simulink model "sample_physmod_load"  (Simulink 6.4)
settings: Solver=ode23tb  StartTime=0.0  StopTime=10.0  RelTol=1e-3
libraries: driveline x5, dc_motor_lib x1
settings Model: LastModifiedBy=roaa

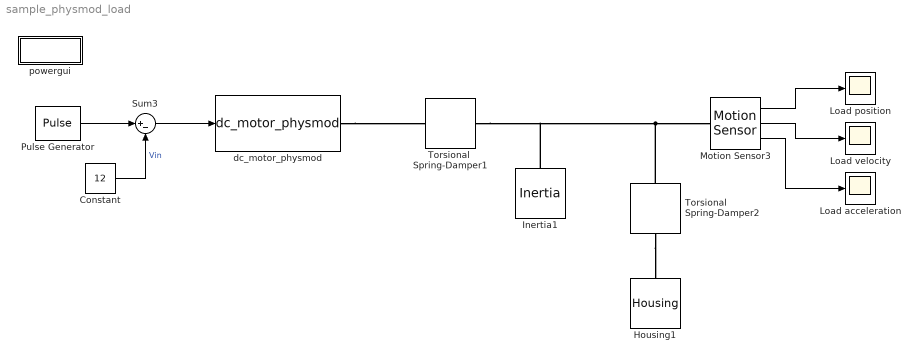
== system sample_physmod_load ==
  Constant : Constant  Value=12  OutDataType=sfix(16)  ConRadixGroup=Use specified scaling  OutScaling=2^0  SampleTime=inf  FramePeriod=inf
  Housing1 : driveline/Solver & Inertias/Housing  Orientation=up  SystemSampleTime=-1
  Inertia1 : driveline/Solver & Inertias/Inertia  Orientation=up  SystemSampleTime=-1  PortType=p1  BlockClass=Inertia  PhysicalDomain=driveline_domain  I=10.07e-6  Ip=[]  Iv=[]  ShowLeft=off  ShowRight=on
  Load acceleration : Scope
  Load position : Scope
      settings: SaveName=ScopeData3
  Load velocity : Scope
  Motion Sensor3 : driveline/Sensors & Actuators/Motion Sensor  SystemSampleTime=-1  Angle=on  x0=0  Velocity=on  Acceleration=on
  Pulse Generator : DiscretePulseGenerator  PulseType=Time based  Amplitude=24  Period=10  PulseWidth=50
  Sum3 : Sum  Inputs=|+-
  Torsional  Spring-Damper1 : driveline/Dynamic Elements/Torsional  Spring-Damper  SystemSampleTime=-1  k=100  c=0.0001  x0=0  Backlash=0
  Torsional  Spring-Damper2 : driveline/Dynamic Elements/Torsional  Spring-Damper  Orientation=up  SystemSampleTime=-1  k=0  c=12e-6  x0=0  Backlash=0
  dc_motor_physmod : dc_motor_lib/dc_motor_physmod  SystemSampleTime=-1  Rm=2.06  Lm=0.000238  Kb=1/((406*2*pi)/60)  Kt=0.0235  Jm=1.07e-6  bm=12e-7
  powergui : Subsystem  AncestorBlock=powerlib/powergui  InitFcn=|  mask(PSB option menu block){SimulationMode=Continuous, SampleTime=0, echomessages=off, x0status=blocks, Frange=[0:2:500], Ylog=off, Xlog=on, ShowGrid=off, save=off, variable=ZData, structure=, ZoomFFT=on, StartTime=0.0, cycles=1, DisplayStyle=1, fundamental=60, FreqAxis=off, MaxFrequency=1000, frequencyindice=1, frequencyindicesteady=1, RmsSteady=1, display=off, Ts=0, frequency=60, methode=off}
      | powerguiblock = gcb;                                        
      | blk = get_param(powerguiblock,'blocks');                    
      | NbBlocks = length(blk);                                     
      | if NbBlocks>2                                               
      | % clean-up:                                                 
      | for m=1:NbBlocks-2                                          
      | delete_block([powerguiblock,'/EquivalentModel',num2str(m)]);
      | end                                                         
      | end
      mask prompts: SimulationMode "General parameter: Simulation Mode"; SampleTime "General parameter: Sample Time"; echomessages "General parameter: Echo  Messages"; x0status "Initial electrical states status"; Frange "Impedance tool: Frequency Range"; Ylog "Impedance tool: Log impedance"; Xlog "Impedance tool: log Frequency"; ShowGrid "Impedance tool: grid"; save "Impedance tool: Save Data To Workspace"; variable "Impedance tool: Variable Name"; structure "Structure Name (PSBFFTSCOPE)"; ZoomFFT "ZoomFFT (PSBFFTSCOPE)"; StartTime "Start Time (PSBFFTSCOPE)"; cycles "Cycles (PSBFFTSCOPE)"; DisplayStyle "Display style (PSBFFTSCOPE)"; fundamental "Fundamental (PSBFFTSCOPE)"; FreqAxis "Frequency Axis (PSBFFTSCOPE)"; MaxFrequency "Max Frequency (PSBFFTSCOPE)"; frequencyindice "Frequency indice  (PSBLOADFLOW)"; frequencyindicesteady "Frequency indice (STEADYSTATE)"; RmsSteady "RMS display (STEADYSTATE)"; display "Display Results"; Ts "Sample time (s):"; frequency "General parameter: phasor frequency"; methode "Phasor simulation"
      mask init:
      | powerlibroot = which('powersysdomain');
      | PSBroot = powerlibroot(1:end-16);
      | %
      | switch SimulationMode
      | 	case 1
      | 		message=sprintf('Continuous');
      | 	case 2
      |         message=sprintf('Discrete,\nTs = %.4g s.',SampleTime);
      | 	case 3
      | 		message=sprintf('Phasors');
      | end
      | if strcmp(bdroot,'powerlib')
      |   message='powergui';
      | end
      | power_initmask();
      settings: CopyFcn=powergui('Copy_Callback',gcb,0,[]);  DeleteFcn=powergui('Copy_Callback',gcb,1,[]);powergui('Close_Callback',gcb,[],[]);  ModelCloseFcn=powergui('Close_Callback',gcb,[],[]);  NameChangeFcn=handles = get_param(gcb,'UserData');if ~isempty(handles);delete(handles.powergui);end
      settings: PreSaveFcn=|
      | %try
      | %close(get_param(gcbh,'userdata'))
      | %end
      | 
      | powergui('Close_Callback',gcb,[],[]);
      settings: OpenFcn=|
      | if (power_openblockproxy ('secondary'))
      | powergui(gcb,'PM')
      | end;
      mask Help: web(psbhelp)
      mask StyleString: popup(Continuous|Discrete|Phasor),edit,checkbox,popup(blocks|steady|zero),edit,checkbox,checkbox,checkbox,checkbox,edit,edit,checkbox,edit,edit,edit,edit,checkbox,edit,edit,edit,edit,checkbox,edit,edit,checkbox
      mask Display: disp(message)
  wires:
  Pulse Generator/1 -> Sum3/1
  Constant/1 -> Sum3/2  "Vin"
  Sum3/1 -> dc_motor_physmod/1
  Motion Sensor3/1 -> Load position/1
  Motion Sensor3/2 -> Load velocity/1
  Motion Sensor3/3 -> Load acceleration/1
  connections:
  dc_motor_physmod/RConn1 -- Torsional  Spring-Damper1/LConn1
  Torsional  Spring-Damper2/LConn1 -- Housing1/RConn1
  Torsional  Spring-Damper1/RConn1 -- Inertia1/RConn1 -- Motion Sensor3/LConn1 -- Torsional  Spring-Damper2/RConn1

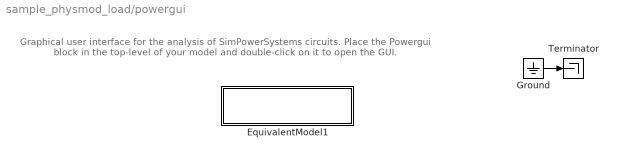
== system sample_physmod_load/powergui ==
  note: Graphical user interface for the analysis of  SimPowerSystems circuits.
      | Place the Powergui block in the top-level of your model and double-click
      | on it to open the GUI.
  EquivalentModel1 : Subsystem
      mask init:
      | SPS = get_param(gcbh,'UserData');
      | if isempty(SPS)
      |     A=0;
      |     B=0;
      |     C=0;
      |     D=0;
      |     x0=0;
      | else
      | 	A=SPS.A;
      |     B=SPS.B;
      |     C=SPS.C;
      |     D=SPS.D;
      |     x0=SPS.x0;
      | end
      mask Display:
      | color('green')
      | disp('EQUIVALENT CIRCUIT')
  Ground : Ground
  Terminator : Terminator
  wires:
  Ground/1 -> Terminator/1

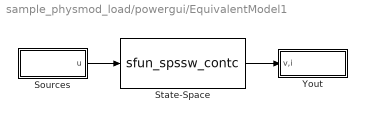
== system sample_physmod_load/powergui/EquivalentModel1 ==
  Sources : Subsystem
  State-Space : S-Function  FunctionName=sfun_spssw_contc  Parameters=A, B, C, D, x0
  Yout : Subsystem
  wires:
  State-Space/1 -> Yout/1(v,i)
  Sources/1(u) -> State-Space/1

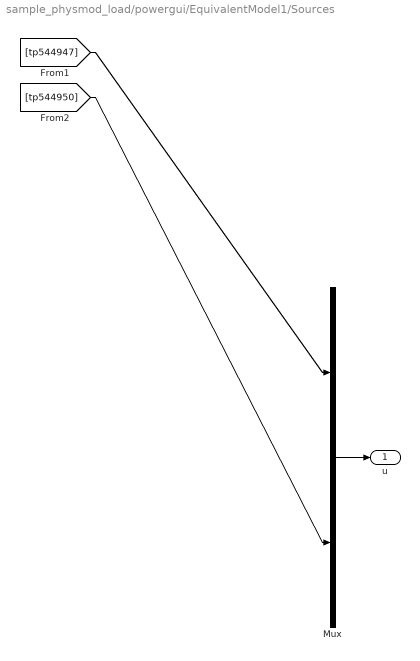
== system sample_physmod_load/powergui/EquivalentModel1/Sources ==
  Mux : Mux  Inputs=[1 1]
  u : Outport
  wires:
  Mux/1 -> u/1
  [tp544947] -> Mux/1
  [tp544950] -> Mux/2

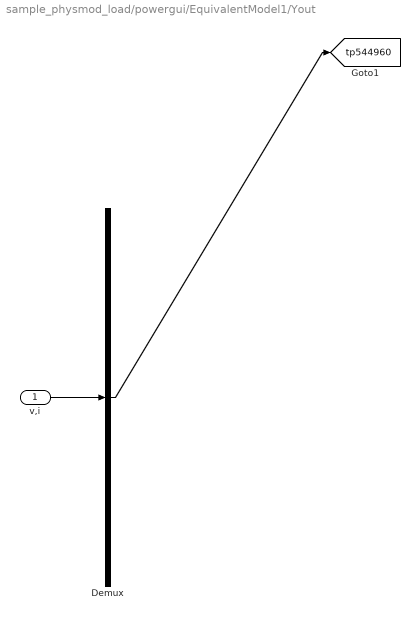
== system sample_physmod_load/powergui/EquivalentModel1/Yout ==
  v,i : Inport
  Demux : Demux  Outputs=1
  tag scope: tp544960=global
  wires:
  v,i/1 -> Demux/1
  Demux/1 -> [tp544960]
